simulink model "elevatorMod"  (R2020a)
settings: Solver=VariableStepAuto  StartTime=0.0  StopTime=inf  RelTol=1e-3
PreLoadFcn:
  | slplc.api.loadDataTypes;
undefined symbols (not defined in the file): BOOL, DINT, INT, slplc
libraries: simulink x1
(part 19 of 39)

== system elevatorMod/PLCControllerSuite/__Logic/Task/Program/__Logic/XIC35/Instruction_Enable ==
  Rung-condition-in : Inport  OutDataTypeStr=BOOL
  Enable : EnablePort
  Logical Operator : Logic  OutDataTypeStr=BOOL
  __CoreVarRead : Subsystem  Tag=CoreVarReadBlock  DisableCoverage=on  TreatAsAtomicUnit=on  mask{PLCBlockType=CoreVarRead}
      mask init:
      | slplc.callbacks.initCoreVariable(gcb, 'read');
      mask Help: web([docroot '/plccoder/ref/__corevarread' '.html']);
      mask DialogControl PLCBlockTitle Prompt: Core Variable Read
  Rung-condition-out : Outport  VectorParamsAs1DForOutWhenUnconnected=off
  wires:
  __CoreVarRead/1(y) -> Logical Operator/2  "DataBit"
  Logical Operator/1 -> Rung-condition-out/1  "Rung-condition-out"
  Rung-condition-in/1 -> Logical Operator/1  "Rung-condition-in"

== system elevatorMod/PLCControllerSuite/__Logic/Task/Program/__Logic/XIC35/RungInOverride ==
  In1 : Inport
  AND : Logic  AllPortsSameDT=off  OutDataTypeStr=boolean
  ForceRungInFalseRead : Subsystem  DisableCoverage=on  TreatAsAtomicUnit=on  mask{PLCLabelTag=_Force_RungIn_False, PLCBlockType=ForceRungInFalseRead}
      mask prompts: PLCLabelTag "Label Tag:"
      mask init:
      | block = gcb;
      | maskObj = Simulink.Mask.get(block);
      | maskObj.Display = sprintf('disp(''%s'');', PLCLabelTag);
      mask Help: web([docroot '/plccoder/ref/forcerunginfalseread' '.html']);
      mask DialogControl PLCBlockTitle Prompt: Force Rung-In False Read
      mask Display: disp('_Force_RungIn_False');
  NOT : Logic  Operator=NOT  IconShape=distinctive  AllPortsSameDT=off  OutDataTypeStr=boolean
  Out1 : Outport  VectorParamsAs1DForOutWhenUnconnected=off
  wires:
  NOT/1 -> AND/1
  ForceRungInFalseRead/1(Out1) -> NOT/1
  In1/1 -> AND/2
  AND/1 -> Out1/1

== system elevatorMod/PLCControllerSuite/__Logic/Task/Program/__Logic/XIC35/__CoreVarRead ==
  DataRead : DataStoreRead  DataStoreName=xxx_PLC_VAR_F2PBHold
  y : Outport  VectorParamsAs1DForOutWhenUnconnected=off
  wires:
  DataRead/1 -> y/1

== system elevatorMod/PLCControllerSuite/__Logic/Task/Program/__Logic/XIC36/BlockEnableRead ==
  __CoreLabelRead : Subsystem  Tag=CoreVarReadBlock  DisableCoverage=on  TreatAsAtomicUnit=on  mask{PLCBlockType=CoreLabelRead}
      mask init:
      | slplc.callbacks.initRoutineLabelRead(gcb);
      mask Help: web([docroot '/plccoder/ref/__corelabelread' '.html']);
      mask DialogControl PLCBlockTitle Prompt: Core Label Read
  Out1 : Outport  VectorParamsAs1DForOutWhenUnconnected=off
  wires:
  __CoreLabelRead/1(Out1) -> Out1/1

== system elevatorMod/PLCControllerSuite/__Logic/Task/Program/__Logic/XIC36/Instruction_Enable ==
  Rung-condition-in : Inport  OutDataTypeStr=BOOL
  Enable : EnablePort
  Logical Operator : Logic  OutDataTypeStr=BOOL
  __CoreVarRead : Subsystem  Tag=CoreVarReadBlock  DisableCoverage=on  TreatAsAtomicUnit=on  mask{PLCBlockType=CoreVarRead}
      mask init:
      | slplc.callbacks.initCoreVariable(gcb, 'read');
      mask Help: web([docroot '/plccoder/ref/__corevarread' '.html']);
      mask DialogControl PLCBlockTitle Prompt: Core Variable Read
  Rung-condition-out : Outport  VectorParamsAs1DForOutWhenUnconnected=off
  wires:
  Rung-condition-in/1 -> Logical Operator/1  "Rung-condition-in"
  Logical Operator/1 -> Rung-condition-out/1  "Rung-condition-out"
  __CoreVarRead/1(y) -> Logical Operator/2  "DataBit"

== system elevatorMod/PLCControllerSuite/__Logic/Task/Program/__Logic/XIC36/RungInOverride ==
  In1 : Inport
  AND : Logic  AllPortsSameDT=off  OutDataTypeStr=boolean
  ForceRungInFalseRead : Subsystem  DisableCoverage=on  TreatAsAtomicUnit=on  mask{PLCLabelTag=_Force_RungIn_False, PLCBlockType=ForceRungInFalseRead}
      mask prompts: PLCLabelTag "Label Tag:"
      mask init:
      | block = gcb;
      | maskObj = Simulink.Mask.get(block);
      | maskObj.Display = sprintf('disp(''%s'');', PLCLabelTag);
      mask Help: web([docroot '/plccoder/ref/forcerunginfalseread' '.html']);
      mask DialogControl PLCBlockTitle Prompt: Force Rung-In False Read
      mask Display: disp('_Force_RungIn_False');
  NOT : Logic  Operator=NOT  IconShape=distinctive  AllPortsSameDT=off  OutDataTypeStr=boolean
  Out1 : Outport  VectorParamsAs1DForOutWhenUnconnected=off
  wires:
  AND/1 -> Out1/1
  In1/1 -> AND/2
  ForceRungInFalseRead/1(Out1) -> NOT/1
  NOT/1 -> AND/1

== system elevatorMod/PLCControllerSuite/__Logic/Task/Program/__Logic/XIC36/__CoreVarRead ==
  DataRead : DataStoreRead  DataStoreName=xxx_PLC_VAR_F3DownBHold
  y : Outport  VectorParamsAs1DForOutWhenUnconnected=off
  wires:
  DataRead/1 -> y/1

== system elevatorMod/PLCControllerSuite/__Logic/Task/Program/__Logic/XIC37/BlockEnableRead ==
  __CoreLabelRead : Subsystem  Tag=CoreVarReadBlock  DisableCoverage=on  TreatAsAtomicUnit=on  mask{PLCBlockType=CoreLabelRead}
      mask init:
      | slplc.callbacks.initRoutineLabelRead(gcb);
      mask Help: web([docroot '/plccoder/ref/__corelabelread' '.html']);
      mask DialogControl PLCBlockTitle Prompt: Core Label Read
  Out1 : Outport  VectorParamsAs1DForOutWhenUnconnected=off
  wires:
  __CoreLabelRead/1(Out1) -> Out1/1

== system elevatorMod/PLCControllerSuite/__Logic/Task/Program/__Logic/XIC37/Instruction_Enable ==
  Rung-condition-in : Inport  OutDataTypeStr=BOOL
  Enable : EnablePort
  Logical Operator : Logic  OutDataTypeStr=BOOL
  __CoreVarRead : Subsystem  Tag=CoreVarReadBlock  DisableCoverage=on  TreatAsAtomicUnit=on  mask{PLCBlockType=CoreVarRead}
      mask init:
      | slplc.callbacks.initCoreVariable(gcb, 'read');
      mask Help: web([docroot '/plccoder/ref/__corevarread' '.html']);
      mask DialogControl PLCBlockTitle Prompt: Core Variable Read
  Rung-condition-out : Outport  VectorParamsAs1DForOutWhenUnconnected=off
  wires:
  Rung-condition-in/1 -> Logical Operator/1  "Rung-condition-in"
  Logical Operator/1 -> Rung-condition-out/1  "Rung-condition-out"
  __CoreVarRead/1(y) -> Logical Operator/2  "DataBit"

== system elevatorMod/PLCControllerSuite/__Logic/Task/Program/__Logic/XIC37/RungInOverride ==
  In1 : Inport
  AND : Logic  AllPortsSameDT=off  OutDataTypeStr=boolean
  ForceRungInFalseRead : Subsystem  DisableCoverage=on  TreatAsAtomicUnit=on  mask{PLCLabelTag=_Force_RungIn_False, PLCBlockType=ForceRungInFalseRead}
      mask prompts: PLCLabelTag "Label Tag:"
      mask init:
      | block = gcb;
      | maskObj = Simulink.Mask.get(block);
      | maskObj.Display = sprintf('disp(''%s'');', PLCLabelTag);
      mask Help: web([docroot '/plccoder/ref/forcerunginfalseread' '.html']);
      mask DialogControl PLCBlockTitle Prompt: Force Rung-In False Read
      mask Display: disp('_Force_RungIn_False');
  NOT : Logic  Operator=NOT  IconShape=distinctive  AllPortsSameDT=off  OutDataTypeStr=boolean
  Out1 : Outport  VectorParamsAs1DForOutWhenUnconnected=off
  wires:
  AND/1 -> Out1/1
  In1/1 -> AND/2
  ForceRungInFalseRead/1(Out1) -> NOT/1
  NOT/1 -> AND/1

== system elevatorMod/PLCControllerSuite/__Logic/Task/Program/__Logic/XIC37/__CoreVarRead ==
  DataRead : DataStoreRead  DataStoreName=xxx_PLC_VAR_F2PBHold
  y : Outport  VectorParamsAs1DForOutWhenUnconnected=off
  wires:
  DataRead/1 -> y/1

== system elevatorMod/PLCControllerSuite/__Logic/Task/Program/__Logic/XIC38/BlockEnableRead ==
  __CoreLabelRead : Subsystem  Tag=CoreVarReadBlock  DisableCoverage=on  TreatAsAtomicUnit=on  mask{PLCBlockType=CoreLabelRead}
      mask init:
      | slplc.callbacks.initRoutineLabelRead(gcb);
      mask Help: web([docroot '/plccoder/ref/__corelabelread' '.html']);
      mask DialogControl PLCBlockTitle Prompt: Core Label Read
  Out1 : Outport  VectorParamsAs1DForOutWhenUnconnected=off
  wires:
  __CoreLabelRead/1(Out1) -> Out1/1

== system elevatorMod/PLCControllerSuite/__Logic/Task/Program/__Logic/XIC38/Instruction_Enable ==
  Rung-condition-in : Inport  OutDataTypeStr=BOOL
  Enable : EnablePort
  Logical Operator : Logic  OutDataTypeStr=BOOL
  __CoreVarRead : Subsystem  Tag=CoreVarReadBlock  DisableCoverage=on  TreatAsAtomicUnit=on  mask{PLCBlockType=CoreVarRead}
      mask init:
      | slplc.callbacks.initCoreVariable(gcb, 'read');
      mask Help: web([docroot '/plccoder/ref/__corevarread' '.html']);
      mask DialogControl PLCBlockTitle Prompt: Core Variable Read
  Rung-condition-out : Outport  VectorParamsAs1DForOutWhenUnconnected=off
  wires:
  __CoreVarRead/1(y) -> Logical Operator/2  "DataBit"
  Logical Operator/1 -> Rung-condition-out/1  "Rung-condition-out"
  Rung-condition-in/1 -> Logical Operator/1  "Rung-condition-in"

== system elevatorMod/PLCControllerSuite/__Logic/Task/Program/__Logic/XIC38/RungInOverride ==
  In1 : Inport
  AND : Logic  AllPortsSameDT=off  OutDataTypeStr=boolean
  ForceRungInFalseRead : Subsystem  DisableCoverage=on  TreatAsAtomicUnit=on  mask{PLCLabelTag=_Force_RungIn_False, PLCBlockType=ForceRungInFalseRead}
      mask prompts: PLCLabelTag "Label Tag:"
      mask init:
      | block = gcb;
      | maskObj = Simulink.Mask.get(block);
      | maskObj.Display = sprintf('disp(''%s'');', PLCLabelTag);
      mask Help: web([docroot '/plccoder/ref/forcerunginfalseread' '.html']);
      mask DialogControl PLCBlockTitle Prompt: Force Rung-In False Read
      mask Display: disp('_Force_RungIn_False');
  NOT : Logic  Operator=NOT  IconShape=distinctive  AllPortsSameDT=off  OutDataTypeStr=boolean
  Out1 : Outport  VectorParamsAs1DForOutWhenUnconnected=off
  wires:
  NOT/1 -> AND/1
  ForceRungInFalseRead/1(Out1) -> NOT/1
  In1/1 -> AND/2
  AND/1 -> Out1/1

== system elevatorMod/PLCControllerSuite/__Logic/Task/Program/__Logic/XIC38/__CoreVarRead ==
  DataRead : DataStoreRead  DataStoreName=xxx_PLC_VAR_MTRON
  y : Outport  VectorParamsAs1DForOutWhenUnconnected=off
  wires:
  DataRead/1 -> y/1

== system elevatorMod/PLCControllerSuite/__Logic/Task/Program/__Logic/XIC39/BlockEnableRead ==
  __CoreLabelRead : Subsystem  Tag=CoreVarReadBlock  DisableCoverage=on  TreatAsAtomicUnit=on  mask{PLCBlockType=CoreLabelRead}
      mask init:
      | slplc.callbacks.initRoutineLabelRead(gcb);
      mask Help: web([docroot '/plccoder/ref/__corelabelread' '.html']);
      mask DialogControl PLCBlockTitle Prompt: Core Label Read
  Out1 : Outport  VectorParamsAs1DForOutWhenUnconnected=off
  wires:
  __CoreLabelRead/1(Out1) -> Out1/1

== system elevatorMod/PLCControllerSuite/__Logic/Task/Program/__Logic/XIC39/Instruction_Enable ==
  Rung-condition-in : Inport  OutDataTypeStr=BOOL
  Enable : EnablePort
  Logical Operator : Logic  OutDataTypeStr=BOOL
  __CoreVarRead : Subsystem  Tag=CoreVarReadBlock  DisableCoverage=on  TreatAsAtomicUnit=on  mask{PLCBlockType=CoreVarRead}
      mask init:
      | slplc.callbacks.initCoreVariable(gcb, 'read');
      mask Help: web([docroot '/plccoder/ref/__corevarread' '.html']);
      mask DialogControl PLCBlockTitle Prompt: Core Variable Read
  Rung-condition-out : Outport  VectorParamsAs1DForOutWhenUnconnected=off
  wires:
  Rung-condition-in/1 -> Logical Operator/1  "Rung-condition-in"
  Logical Operator/1 -> Rung-condition-out/1  "Rung-condition-out"
  __CoreVarRead/1(y) -> Logical Operator/2  "DataBit"

== system elevatorMod/PLCControllerSuite/__Logic/Task/Program/__Logic/XIC39/RungInOverride ==
  In1 : Inport
  AND : Logic  AllPortsSameDT=off  OutDataTypeStr=boolean
  ForceRungInFalseRead : Subsystem  DisableCoverage=on  TreatAsAtomicUnit=on  mask{PLCLabelTag=_Force_RungIn_False, PLCBlockType=ForceRungInFalseRead}
      mask prompts: PLCLabelTag "Label Tag:"
      mask init:
      | block = gcb;
      | maskObj = Simulink.Mask.get(block);
      | maskObj.Display = sprintf('disp(''%s'');', PLCLabelTag);
      mask Help: web([docroot '/plccoder/ref/forcerunginfalseread' '.html']);
      mask DialogControl PLCBlockTitle Prompt: Force Rung-In False Read
      mask Display: disp('_Force_RungIn_False');
  NOT : Logic  Operator=NOT  IconShape=distinctive  AllPortsSameDT=off  OutDataTypeStr=boolean
  Out1 : Outport  VectorParamsAs1DForOutWhenUnconnected=off
  wires:
  AND/1 -> Out1/1
  In1/1 -> AND/2
  ForceRungInFalseRead/1(Out1) -> NOT/1
  NOT/1 -> AND/1

== system elevatorMod/PLCControllerSuite/__Logic/Task/Program/__Logic/XIC39/__CoreVarRead ==
  DataRead : DataStoreRead  DataStoreName=xxx_PLC_VAR_RMPUPTRG
  y : Outport  VectorParamsAs1DForOutWhenUnconnected=off
  wires:
  DataRead/1 -> y/1

== system elevatorMod/PLCControllerSuite/__Logic/Task/Program/__Logic/XIC4/BlockEnableRead ==
  __CoreLabelRead : Subsystem  Tag=CoreVarReadBlock  DisableCoverage=on  TreatAsAtomicUnit=on  mask{PLCBlockType=CoreLabelRead}
      mask init:
      | slplc.callbacks.initRoutineLabelRead(gcb);
      mask Help: web([docroot '/plccoder/ref/__corelabelread' '.html']);
      mask DialogControl PLCBlockTitle Prompt: Core Label Read
  Out1 : Outport  VectorParamsAs1DForOutWhenUnconnected=off
  wires:
  __CoreLabelRead/1(Out1) -> Out1/1

== system elevatorMod/PLCControllerSuite/__Logic/Task/Program/__Logic/XIC4/Instruction_Enable ==
  Rung-condition-in : Inport  OutDataTypeStr=BOOL
  Enable : EnablePort
  Logical Operator : Logic  OutDataTypeStr=BOOL
  __CoreVarRead : Subsystem  Tag=CoreVarReadBlock  DisableCoverage=on  TreatAsAtomicUnit=on  mask{PLCBlockType=CoreVarRead}
      mask init:
      | slplc.callbacks.initCoreVariable(gcb, 'read');
      mask Help: web([docroot '/plccoder/ref/__corevarread' '.html']);
      mask DialogControl PLCBlockTitle Prompt: Core Variable Read
  Rung-condition-out : Outport  VectorParamsAs1DForOutWhenUnconnected=off
  wires:
  Rung-condition-in/1 -> Logical Operator/1  "Rung-condition-in"
  Logical Operator/1 -> Rung-condition-out/1  "Rung-condition-out"
  __CoreVarRead/1(y) -> Logical Operator/2  "DataBit"

== system elevatorMod/PLCControllerSuite/__Logic/Task/Program/__Logic/XIC4/RungInOverride ==
  In1 : Inport
  AND : Logic  AllPortsSameDT=off  OutDataTypeStr=boolean
  ForceRungInFalseRead : Subsystem  DisableCoverage=on  TreatAsAtomicUnit=on  mask{PLCLabelTag=_Force_RungIn_False, PLCBlockType=ForceRungInFalseRead}
      mask prompts: PLCLabelTag "Label Tag:"
      mask init:
      | block = gcb;
      | maskObj = Simulink.Mask.get(block);
      | maskObj.Display = sprintf('disp(''%s'');', PLCLabelTag);
      mask Help: web([docroot '/plccoder/ref/forcerunginfalseread' '.html']);
      mask DialogControl PLCBlockTitle Prompt: Force Rung-In False Read
      mask Display: disp('_Force_RungIn_False');
  NOT : Logic  Operator=NOT  IconShape=distinctive  AllPortsSameDT=off  OutDataTypeStr=boolean
  Out1 : Outport  VectorParamsAs1DForOutWhenUnconnected=off
  wires:
  AND/1 -> Out1/1
  In1/1 -> AND/2
  ForceRungInFalseRead/1(Out1) -> NOT/1
  NOT/1 -> AND/1

== system elevatorMod/PLCControllerSuite/__Logic/Task/Program/__Logic/XIC4/__CoreVarRead ==
  DataRead : DataStoreRead  DataStoreName=xxx_PLC_VAR_F1PBHold
  y : Outport  VectorParamsAs1DForOutWhenUnconnected=off
  wires:
  DataRead/1 -> y/1

== system elevatorMod/PLCControllerSuite/__Logic/Task/Program/__Logic/XIC40/BlockEnableRead ==
  __CoreLabelRead : Subsystem  Tag=CoreVarReadBlock  DisableCoverage=on  TreatAsAtomicUnit=on  mask{PLCBlockType=CoreLabelRead}
      mask init:
      | slplc.callbacks.initRoutineLabelRead(gcb);
      mask Help: web([docroot '/plccoder/ref/__corelabelread' '.html']);
      mask DialogControl PLCBlockTitle Prompt: Core Label Read
  Out1 : Outport  VectorParamsAs1DForOutWhenUnconnected=off
  wires:
  __CoreLabelRead/1(Out1) -> Out1/1

== system elevatorMod/PLCControllerSuite/__Logic/Task/Program/__Logic/XIC40/Instruction_Enable ==
  Rung-condition-in : Inport  OutDataTypeStr=BOOL
  Enable : EnablePort
  Logical Operator : Logic  OutDataTypeStr=BOOL
  __CoreVarRead : Subsystem  Tag=CoreVarReadBlock  DisableCoverage=on  TreatAsAtomicUnit=on  mask{PLCBlockType=CoreVarRead}
      mask init:
      | slplc.callbacks.initCoreVariable(gcb, 'read');
      mask Help: web([docroot '/plccoder/ref/__corevarread' '.html']);
      mask DialogControl PLCBlockTitle Prompt: Core Variable Read
  Rung-condition-out : Outport  VectorParamsAs1DForOutWhenUnconnected=off
  wires:
  __CoreVarRead/1(y) -> Logical Operator/2  "DataBit"
  Logical Operator/1 -> Rung-condition-out/1  "Rung-condition-out"
  Rung-condition-in/1 -> Logical Operator/1  "Rung-condition-in"

== system elevatorMod/PLCControllerSuite/__Logic/Task/Program/__Logic/XIC40/RungInOverride ==
  In1 : Inport
  AND : Logic  AllPortsSameDT=off  OutDataTypeStr=boolean
  ForceRungInFalseRead : Subsystem  DisableCoverage=on  TreatAsAtomicUnit=on  mask{PLCLabelTag=_Force_RungIn_False, PLCBlockType=ForceRungInFalseRead}
      mask prompts: PLCLabelTag "Label Tag:"
      mask init:
      | block = gcb;
      | maskObj = Simulink.Mask.get(block);
      | maskObj.Display = sprintf('disp(''%s'');', PLCLabelTag);
      mask Help: web([docroot '/plccoder/ref/forcerunginfalseread' '.html']);
      mask DialogControl PLCBlockTitle Prompt: Force Rung-In False Read
      mask Display: disp('_Force_RungIn_False');
  NOT : Logic  Operator=NOT  IconShape=distinctive  AllPortsSameDT=off  OutDataTypeStr=boolean
  Out1 : Outport  VectorParamsAs1DForOutWhenUnconnected=off
  wires:
  NOT/1 -> AND/1
  ForceRungInFalseRead/1(Out1) -> NOT/1
  In1/1 -> AND/2
  AND/1 -> Out1/1

== system elevatorMod/PLCControllerSuite/__Logic/Task/Program/__Logic/XIC40/__CoreVarRead ==
  DataRead : DataStoreRead  DataStoreName=xxx_PLC_VAR_RMPUP
  y : Outport  VectorParamsAs1DForOutWhenUnconnected=off
  wires:
  DataRead/1 -> y/1

== system elevatorMod/PLCControllerSuite/__Logic/Task/Program/__Logic/XIC41/BlockEnableRead ==
  __CoreLabelRead : Subsystem  Tag=CoreVarReadBlock  DisableCoverage=on  TreatAsAtomicUnit=on  mask{PLCBlockType=CoreLabelRead}
      mask init:
      | slplc.callbacks.initRoutineLabelRead(gcb);
      mask Help: web([docroot '/plccoder/ref/__corelabelread' '.html']);
      mask DialogControl PLCBlockTitle Prompt: Core Label Read
  Out1 : Outport  VectorParamsAs1DForOutWhenUnconnected=off
  wires:
  __CoreLabelRead/1(Out1) -> Out1/1

== system elevatorMod/PLCControllerSuite/__Logic/Task/Program/__Logic/XIC41/Instruction_Enable ==
  Rung-condition-in : Inport  OutDataTypeStr=BOOL
  Enable : EnablePort
  Logical Operator : Logic  OutDataTypeStr=BOOL
  __CoreVarRead : Subsystem  Tag=CoreVarReadBlock  DisableCoverage=on  TreatAsAtomicUnit=on  mask{PLCBlockType=CoreVarRead}
      mask init:
      | slplc.callbacks.initCoreVariable(gcb, 'read');
      mask Help: web([docroot '/plccoder/ref/__corevarread' '.html']);
      mask DialogControl PLCBlockTitle Prompt: Core Variable Read
  Rung-condition-out : Outport  VectorParamsAs1DForOutWhenUnconnected=off
  wires:
  __CoreVarRead/1(y) -> Logical Operator/2  "DataBit"
  Logical Operator/1 -> Rung-condition-out/1  "Rung-condition-out"
  Rung-condition-in/1 -> Logical Operator/1  "Rung-condition-in"

== system elevatorMod/PLCControllerSuite/__Logic/Task/Program/__Logic/XIC41/RungInOverride ==
  In1 : Inport
  AND : Logic  AllPortsSameDT=off  OutDataTypeStr=boolean
  ForceRungInFalseRead : Subsystem  DisableCoverage=on  TreatAsAtomicUnit=on  mask{PLCLabelTag=_Force_RungIn_False, PLCBlockType=ForceRungInFalseRead}
      mask prompts: PLCLabelTag "Label Tag:"
      mask init:
      | block = gcb;
      | maskObj = Simulink.Mask.get(block);
      | maskObj.Display = sprintf('disp(''%s'');', PLCLabelTag);
      mask Help: web([docroot '/plccoder/ref/forcerunginfalseread' '.html']);
      mask DialogControl PLCBlockTitle Prompt: Force Rung-In False Read
      mask Display: disp('_Force_RungIn_False');
  NOT : Logic  Operator=NOT  IconShape=distinctive  AllPortsSameDT=off  OutDataTypeStr=boolean
  Out1 : Outport  VectorParamsAs1DForOutWhenUnconnected=off
  wires:
  NOT/1 -> AND/1
  ForceRungInFalseRead/1(Out1) -> NOT/1
  In1/1 -> AND/2
  AND/1 -> Out1/1

== system elevatorMod/PLCControllerSuite/__Logic/Task/Program/__Logic/XIC41/__CoreVarRead ==
  DataRead : DataStoreRead  DataStoreName=xxx_PLC_VAR_SENCHK
  y : Outport  VectorParamsAs1DForOutWhenUnconnected=off
  wires:
  DataRead/1 -> y/1

== system elevatorMod/PLCControllerSuite/__Logic/Task/Program/__Logic/XIC42/BlockEnableRead ==
  __CoreLabelRead : Subsystem  Tag=CoreVarReadBlock  DisableCoverage=on  TreatAsAtomicUnit=on  mask{PLCBlockType=CoreLabelRead}
      mask init:
      | slplc.callbacks.initRoutineLabelRead(gcb);
      mask Help: web([docroot '/plccoder/ref/__corelabelread' '.html']);
      mask DialogControl PLCBlockTitle Prompt: Core Label Read
  Out1 : Outport  VectorParamsAs1DForOutWhenUnconnected=off
  wires:
  __CoreLabelRead/1(Out1) -> Out1/1

== system elevatorMod/PLCControllerSuite/__Logic/Task/Program/__Logic/XIC42/Instruction_Enable ==
  Rung-condition-in : Inport  OutDataTypeStr=BOOL
  Enable : EnablePort
  Logical Operator : Logic  OutDataTypeStr=BOOL
  __CoreVarRead : Subsystem  Tag=CoreVarReadBlock  DisableCoverage=on  TreatAsAtomicUnit=on  mask{PLCBlockType=CoreVarRead}
      mask init:
      | slplc.callbacks.initCoreVariable(gcb, 'read');
      mask Help: web([docroot '/plccoder/ref/__corevarread' '.html']);
      mask DialogControl PLCBlockTitle Prompt: Core Variable Read
  Rung-condition-out : Outport  VectorParamsAs1DForOutWhenUnconnected=off
  wires:
  Rung-condition-in/1 -> Logical Operator/1  "Rung-condition-in"
  Logical Operator/1 -> Rung-condition-out/1  "Rung-condition-out"
  __CoreVarRead/1(y) -> Logical Operator/2  "DataBit"

== system elevatorMod/PLCControllerSuite/__Logic/Task/Program/__Logic/XIC42/RungInOverride ==
  In1 : Inport
  AND : Logic  AllPortsSameDT=off  OutDataTypeStr=boolean
  ForceRungInFalseRead : Subsystem  DisableCoverage=on  TreatAsAtomicUnit=on  mask{PLCLabelTag=_Force_RungIn_False, PLCBlockType=ForceRungInFalseRead}
      mask prompts: PLCLabelTag "Label Tag:"
      mask init:
      | block = gcb;
      | maskObj = Simulink.Mask.get(block);
      | maskObj.Display = sprintf('disp(''%s'');', PLCLabelTag);
      mask Help: web([docroot '/plccoder/ref/forcerunginfalseread' '.html']);
      mask DialogControl PLCBlockTitle Prompt: Force Rung-In False Read
      mask Display: disp('_Force_RungIn_False');
  NOT : Logic  Operator=NOT  IconShape=distinctive  AllPortsSameDT=off  OutDataTypeStr=boolean
  Out1 : Outport  VectorParamsAs1DForOutWhenUnconnected=off
  wires:
  AND/1 -> Out1/1
  In1/1 -> AND/2
  ForceRungInFalseRead/1(Out1) -> NOT/1
  NOT/1 -> AND/1

== system elevatorMod/PLCControllerSuite/__Logic/Task/Program/__Logic/XIC42/__CoreVarRead ==
  DataRead : DataStoreRead  DataStoreName=xxx_PLC_VAR_StartHold
  y : Outport  VectorParamsAs1DForOutWhenUnconnected=off
  wires:
  DataRead/1 -> y/1

== system elevatorMod/PLCControllerSuite/__Logic/Task/Program/__Logic/XIC43/BlockEnableRead ==
  __CoreLabelRead : Subsystem  Tag=CoreVarReadBlock  DisableCoverage=on  TreatAsAtomicUnit=on  mask{PLCBlockType=CoreLabelRead}
      mask init:
      | slplc.callbacks.initRoutineLabelRead(gcb);
      mask Help: web([docroot '/plccoder/ref/__corelabelread' '.html']);
      mask DialogControl PLCBlockTitle Prompt: Core Label Read
  Out1 : Outport  VectorParamsAs1DForOutWhenUnconnected=off
  wires:
  __CoreLabelRead/1(Out1) -> Out1/1

== system elevatorMod/PLCControllerSuite/__Logic/Task/Program/__Logic/XIC43/Instruction_Enable ==
  Rung-condition-in : Inport  OutDataTypeStr=BOOL
  Enable : EnablePort
  Logical Operator : Logic  OutDataTypeStr=BOOL
  __CoreVarRead : Subsystem  Tag=CoreVarReadBlock  DisableCoverage=on  TreatAsAtomicUnit=on  mask{PLCBlockType=CoreVarRead}
      mask init:
      | slplc.callbacks.initCoreVariable(gcb, 'read');
      mask Help: web([docroot '/plccoder/ref/__corevarread' '.html']);
      mask DialogControl PLCBlockTitle Prompt: Core Variable Read
  Rung-condition-out : Outport  VectorParamsAs1DForOutWhenUnconnected=off
  wires:
  Rung-condition-in/1 -> Logical Operator/1  "Rung-condition-in"
  Logical Operator/1 -> Rung-condition-out/1  "Rung-condition-out"
  __CoreVarRead/1(y) -> Logical Operator/2  "DataBit"

== system elevatorMod/PLCControllerSuite/__Logic/Task/Program/__Logic/XIC43/RungInOverride ==
  In1 : Inport
  AND : Logic  AllPortsSameDT=off  OutDataTypeStr=boolean
  ForceRungInFalseRead : Subsystem  DisableCoverage=on  TreatAsAtomicUnit=on  mask{PLCLabelTag=_Force_RungIn_False, PLCBlockType=ForceRungInFalseRead}
      mask prompts: PLCLabelTag "Label Tag:"
      mask init:
      | block = gcb;
      | maskObj = Simulink.Mask.get(block);
      | maskObj.Display = sprintf('disp(''%s'');', PLCLabelTag);
      mask Help: web([docroot '/plccoder/ref/forcerunginfalseread' '.html']);
      mask DialogControl PLCBlockTitle Prompt: Force Rung-In False Read
      mask Display: disp('_Force_RungIn_False');
  NOT : Logic  Operator=NOT  IconShape=distinctive  AllPortsSameDT=off  OutDataTypeStr=boolean
  Out1 : Outport  VectorParamsAs1DForOutWhenUnconnected=off
  wires:
  AND/1 -> Out1/1
  In1/1 -> AND/2
  ForceRungInFalseRead/1(Out1) -> NOT/1
  NOT/1 -> AND/1

== system elevatorMod/PLCControllerSuite/__Logic/Task/Program/__Logic/XIC43/__CoreVarRead ==
  DataRead : DataStoreRead  DataStoreName=xxx_PLC_VAR_TempS3LUp
  y : Outport  VectorParamsAs1DForOutWhenUnconnected=off
  wires:
  DataRead/1 -> y/1

== system elevatorMod/PLCControllerSuite/__Logic/Task/Program/__Logic/XIC44/BlockEnableRead ==
  __CoreLabelRead : Subsystem  Tag=CoreVarReadBlock  DisableCoverage=on  TreatAsAtomicUnit=on  mask{PLCBlockType=CoreLabelRead}
      mask init:
      | slplc.callbacks.initRoutineLabelRead(gcb);
      mask Help: web([docroot '/plccoder/ref/__corelabelread' '.html']);
      mask DialogControl PLCBlockTitle Prompt: Core Label Read
  Out1 : Outport  VectorParamsAs1DForOutWhenUnconnected=off
  wires:
  __CoreLabelRead/1(Out1) -> Out1/1

== system elevatorMod/PLCControllerSuite/__Logic/Task/Program/__Logic/XIC44/Instruction_Enable ==
  Rung-condition-in : Inport  OutDataTypeStr=BOOL
  Enable : EnablePort
  Logical Operator : Logic  OutDataTypeStr=BOOL
  __CoreVarRead : Subsystem  Tag=CoreVarReadBlock  DisableCoverage=on  TreatAsAtomicUnit=on  mask{PLCBlockType=CoreVarRead}
      mask init:
      | slplc.callbacks.initCoreVariable(gcb, 'read');
      mask Help: web([docroot '/plccoder/ref/__corevarread' '.html']);
      mask DialogControl PLCBlockTitle Prompt: Core Variable Read
  Rung-condition-out : Outport  VectorParamsAs1DForOutWhenUnconnected=off
  wires:
  __CoreVarRead/1(y) -> Logical Operator/2  "DataBit"
  Logical Operator/1 -> Rung-condition-out/1  "Rung-condition-out"
  Rung-condition-in/1 -> Logical Operator/1  "Rung-condition-in"

== system elevatorMod/PLCControllerSuite/__Logic/Task/Program/__Logic/XIC44/RungInOverride ==
  In1 : Inport
  AND : Logic  AllPortsSameDT=off  OutDataTypeStr=boolean
  ForceRungInFalseRead : Subsystem  DisableCoverage=on  TreatAsAtomicUnit=on  mask{PLCLabelTag=_Force_RungIn_False, PLCBlockType=ForceRungInFalseRead}
      mask prompts: PLCLabelTag "Label Tag:"
      mask init:
      | block = gcb;
      | maskObj = Simulink.Mask.get(block);
      | maskObj.Display = sprintf('disp(''%s'');', PLCLabelTag);
      mask Help: web([docroot '/plccoder/ref/forcerunginfalseread' '.html']);
      mask DialogControl PLCBlockTitle Prompt: Force Rung-In False Read
      mask Display: disp('_Force_RungIn_False');
  NOT : Logic  Operator=NOT  IconShape=distinctive  AllPortsSameDT=off  OutDataTypeStr=boolean
  Out1 : Outport  VectorParamsAs1DForOutWhenUnconnected=off
  wires:
  NOT/1 -> AND/1
  ForceRungInFalseRead/1(Out1) -> NOT/1
  In1/1 -> AND/2
  AND/1 -> Out1/1

== system elevatorMod/PLCControllerSuite/__Logic/Task/Program/__Logic/XIC44/__CoreVarRead ==
  DataRead : DataStoreRead  DataStoreName=xxx_PLC_VAR_MemoryGoUp
  y : Outport  VectorParamsAs1DForOutWhenUnconnected=off
  wires:
  DataRead/1 -> y/1

== system elevatorMod/PLCControllerSuite/__Logic/Task/Program/__Logic/XIC45/BlockEnableRead ==
  __CoreLabelRead : Subsystem  Tag=CoreVarReadBlock  DisableCoverage=on  TreatAsAtomicUnit=on  mask{PLCBlockType=CoreLabelRead}
      mask init:
      | slplc.callbacks.initRoutineLabelRead(gcb);
      mask Help: web([docroot '/plccoder/ref/__corelabelread' '.html']);
      mask DialogControl PLCBlockTitle Prompt: Core Label Read
  Out1 : Outport  VectorParamsAs1DForOutWhenUnconnected=off
  wires:
  __CoreLabelRead/1(Out1) -> Out1/1

== system elevatorMod/PLCControllerSuite/__Logic/Task/Program/__Logic/XIC45/Instruction_Enable ==
  Rung-condition-in : Inport  OutDataTypeStr=BOOL
  Enable : EnablePort
  Logical Operator : Logic  OutDataTypeStr=BOOL
  __CoreVarRead : Subsystem  Tag=CoreVarReadBlock  DisableCoverage=on  TreatAsAtomicUnit=on  mask{PLCBlockType=CoreVarRead}
      mask init:
      | slplc.callbacks.initCoreVariable(gcb, 'read');
      mask Help: web([docroot '/plccoder/ref/__corevarread' '.html']);
      mask DialogControl PLCBlockTitle Prompt: Core Variable Read
  Rung-condition-out : Outport  VectorParamsAs1DForOutWhenUnconnected=off
  wires:
  Rung-condition-in/1 -> Logical Operator/1  "Rung-condition-in"
  Logical Operator/1 -> Rung-condition-out/1  "Rung-condition-out"
  __CoreVarRead/1(y) -> Logical Operator/2  "DataBit"

== system elevatorMod/PLCControllerSuite/__Logic/Task/Program/__Logic/XIC45/RungInOverride ==
  In1 : Inport
  AND : Logic  AllPortsSameDT=off  OutDataTypeStr=boolean
  ForceRungInFalseRead : Subsystem  DisableCoverage=on  TreatAsAtomicUnit=on  mask{PLCLabelTag=_Force_RungIn_False, PLCBlockType=ForceRungInFalseRead}
      mask prompts: PLCLabelTag "Label Tag:"
      mask init:
      | block = gcb;
      | maskObj = Simulink.Mask.get(block);
      | maskObj.Display = sprintf('disp(''%s'');', PLCLabelTag);
      mask Help: web([docroot '/plccoder/ref/forcerunginfalseread' '.html']);
      mask DialogControl PLCBlockTitle Prompt: Force Rung-In False Read
      mask Display: disp('_Force_RungIn_False');
  NOT : Logic  Operator=NOT  IconShape=distinctive  AllPortsSameDT=off  OutDataTypeStr=boolean
  Out1 : Outport  VectorParamsAs1DForOutWhenUnconnected=off
  wires:
  AND/1 -> Out1/1
  In1/1 -> AND/2
  ForceRungInFalseRead/1(Out1) -> NOT/1
  NOT/1 -> AND/1

== system elevatorMod/PLCControllerSuite/__Logic/Task/Program/__Logic/XIC45/__CoreVarRead ==
  DataRead : DataStoreRead  DataStoreName=xxx_PLC_VAR_StartHold
  y : Outport  VectorParamsAs1DForOutWhenUnconnected=off
  wires:
  DataRead/1 -> y/1

== system elevatorMod/PLCControllerSuite/__Logic/Task/Program/__Logic/XIC46/BlockEnableRead ==
  __CoreLabelRead : Subsystem  Tag=CoreVarReadBlock  DisableCoverage=on  TreatAsAtomicUnit=on  mask{PLCBlockType=CoreLabelRead}
      mask init:
      | slplc.callbacks.initRoutineLabelRead(gcb);
      mask Help: web([docroot '/plccoder/ref/__corelabelread' '.html']);
      mask DialogControl PLCBlockTitle Prompt: Core Label Read
  Out1 : Outport  VectorParamsAs1DForOutWhenUnconnected=off
  wires:
  __CoreLabelRead/1(Out1) -> Out1/1

== system elevatorMod/PLCControllerSuite/__Logic/Task/Program/__Logic/XIC46/Instruction_Enable ==
  Rung-condition-in : Inport  OutDataTypeStr=BOOL
  Enable : EnablePort
  Logical Operator : Logic  OutDataTypeStr=BOOL
  __CoreVarRead : Subsystem  Tag=CoreVarReadBlock  DisableCoverage=on  TreatAsAtomicUnit=on  mask{PLCBlockType=CoreVarRead}
      mask init:
      | slplc.callbacks.initCoreVariable(gcb, 'read');
      mask Help: web([docroot '/plccoder/ref/__corevarread' '.html']);
      mask DialogControl PLCBlockTitle Prompt: Core Variable Read
  Rung-condition-out : Outport  VectorParamsAs1DForOutWhenUnconnected=off
  wires:
  __CoreVarRead/1(y) -> Logical Operator/2  "DataBit"
  Logical Operator/1 -> Rung-condition-out/1  "Rung-condition-out"
  Rung-condition-in/1 -> Logical Operator/1  "Rung-condition-in"

== system elevatorMod/PLCControllerSuite/__Logic/Task/Program/__Logic/XIC46/RungInOverride ==
  In1 : Inport
  AND : Logic  AllPortsSameDT=off  OutDataTypeStr=boolean
  ForceRungInFalseRead : Subsystem  DisableCoverage=on  TreatAsAtomicUnit=on  mask{PLCLabelTag=_Force_RungIn_False, PLCBlockType=ForceRungInFalseRead}
      mask prompts: PLCLabelTag "Label Tag:"
      mask init:
      | block = gcb;
      | maskObj = Simulink.Mask.get(block);
      | maskObj.Display = sprintf('disp(''%s'');', PLCLabelTag);
      mask Help: web([docroot '/plccoder/ref/forcerunginfalseread' '.html']);
      mask DialogControl PLCBlockTitle Prompt: Force Rung-In False Read
      mask Display: disp('_Force_RungIn_False');
  NOT : Logic  Operator=NOT  IconShape=distinctive  AllPortsSameDT=off  OutDataTypeStr=boolean
  Out1 : Outport  VectorParamsAs1DForOutWhenUnconnected=off
  wires:
  NOT/1 -> AND/1
  ForceRungInFalseRead/1(Out1) -> NOT/1
  In1/1 -> AND/2
  AND/1 -> Out1/1

== system elevatorMod/PLCControllerSuite/__Logic/Task/Program/__Logic/XIC46/__CoreVarRead ==
  DataRead : DataStoreRead  DataStoreName=xxx_PLC_VAR_S1H
  y : Outport  VectorParamsAs1DForOutWhenUnconnected=off
  wires:
  DataRead/1 -> y/1

== system elevatorMod/PLCControllerSuite/__Logic/Task/Program/__Logic/XIC47/BlockEnableRead ==
  __CoreLabelRead : Subsystem  Tag=CoreVarReadBlock  DisableCoverage=on  TreatAsAtomicUnit=on  mask{PLCBlockType=CoreLabelRead}
      mask init:
      | slplc.callbacks.initRoutineLabelRead(gcb);
      mask Help: web([docroot '/plccoder/ref/__corelabelread' '.html']);
      mask DialogControl PLCBlockTitle Prompt: Core Label Read
  Out1 : Outport  VectorParamsAs1DForOutWhenUnconnected=off
  wires:
  __CoreLabelRead/1(Out1) -> Out1/1

== system elevatorMod/PLCControllerSuite/__Logic/Task/Program/__Logic/XIC47/Instruction_Enable ==
  Rung-condition-in : Inport  OutDataTypeStr=BOOL
  Enable : EnablePort
  Logical Operator : Logic  OutDataTypeStr=BOOL
  __CoreVarRead : Subsystem  Tag=CoreVarReadBlock  DisableCoverage=on  TreatAsAtomicUnit=on  mask{PLCBlockType=CoreVarRead}
      mask init:
      | slplc.callbacks.initCoreVariable(gcb, 'read');
      mask Help: web([docroot '/plccoder/ref/__corevarread' '.html']);
      mask DialogControl PLCBlockTitle Prompt: Core Variable Read
  Rung-condition-out : Outport  VectorParamsAs1DForOutWhenUnconnected=off
  wires:
  Rung-condition-in/1 -> Logical Operator/1  "Rung-condition-in"
  Logical Operator/1 -> Rung-condition-out/1  "Rung-condition-out"
  __CoreVarRead/1(y) -> Logical Operator/2  "DataBit"

== system elevatorMod/PLCControllerSuite/__Logic/Task/Program/__Logic/XIC47/RungInOverride ==
  In1 : Inport
  AND : Logic  AllPortsSameDT=off  OutDataTypeStr=boolean
  ForceRungInFalseRead : Subsystem  DisableCoverage=on  TreatAsAtomicUnit=on  mask{PLCLabelTag=_Force_RungIn_False, PLCBlockType=ForceRungInFalseRead}
      mask prompts: PLCLabelTag "Label Tag:"
      mask init:
      | block = gcb;
      | maskObj = Simulink.Mask.get(block);
      | maskObj.Display = sprintf('disp(''%s'');', PLCLabelTag);
      mask Help: web([docroot '/plccoder/ref/forcerunginfalseread' '.html']);
      mask DialogControl PLCBlockTitle Prompt: Force Rung-In False Read
      mask Display: disp('_Force_RungIn_False');
  NOT : Logic  Operator=NOT  IconShape=distinctive  AllPortsSameDT=off  OutDataTypeStr=boolean
  Out1 : Outport  VectorParamsAs1DForOutWhenUnconnected=off
  wires:
  AND/1 -> Out1/1
  In1/1 -> AND/2
  ForceRungInFalseRead/1(Out1) -> NOT/1
  NOT/1 -> AND/1

== system elevatorMod/PLCControllerSuite/__Logic/Task/Program/__Logic/XIC47/__CoreVarRead ==
  DataRead : DataStoreRead  DataStoreName=xxx_PLC_VAR_S2L
  y : Outport  VectorParamsAs1DForOutWhenUnconnected=off
  wires:
  DataRead/1 -> y/1

== system elevatorMod/PLCControllerSuite/__Logic/Task/Program/__Logic/XIC48/BlockEnableRead ==
  __CoreLabelRead : Subsystem  Tag=CoreVarReadBlock  DisableCoverage=on  TreatAsAtomicUnit=on  mask{PLCBlockType=CoreLabelRead}
      mask init:
      | slplc.callbacks.initRoutineLabelRead(gcb);
      mask Help: web([docroot '/plccoder/ref/__corelabelread' '.html']);
      mask DialogControl PLCBlockTitle Prompt: Core Label Read
  Out1 : Outport  VectorParamsAs1DForOutWhenUnconnected=off
  wires:
  __CoreLabelRead/1(Out1) -> Out1/1

== system elevatorMod/PLCControllerSuite/__Logic/Task/Program/__Logic/XIC48/Instruction_Enable ==
  Rung-condition-in : Inport  OutDataTypeStr=BOOL
  Enable : EnablePort
  Logical Operator : Logic  OutDataTypeStr=BOOL
  __CoreVarRead : Subsystem  Tag=CoreVarReadBlock  DisableCoverage=on  TreatAsAtomicUnit=on  mask{PLCBlockType=CoreVarRead}
      mask init:
      | slplc.callbacks.initCoreVariable(gcb, 'read');
      mask Help: web([docroot '/plccoder/ref/__corevarread' '.html']);
      mask DialogControl PLCBlockTitle Prompt: Core Variable Read
  Rung-condition-out : Outport  VectorParamsAs1DForOutWhenUnconnected=off
  wires:
  Rung-condition-in/1 -> Logical Operator/1  "Rung-condition-in"
  Logical Operator/1 -> Rung-condition-out/1  "Rung-condition-out"
  __CoreVarRead/1(y) -> Logical Operator/2  "DataBit"

== system elevatorMod/PLCControllerSuite/__Logic/Task/Program/__Logic/XIC48/RungInOverride ==
  In1 : Inport
  AND : Logic  AllPortsSameDT=off  OutDataTypeStr=boolean
  ForceRungInFalseRead : Subsystem  DisableCoverage=on  TreatAsAtomicUnit=on  mask{PLCLabelTag=_Force_RungIn_False, PLCBlockType=ForceRungInFalseRead}
      mask prompts: PLCLabelTag "Label Tag:"
      mask init:
      | block = gcb;
      | maskObj = Simulink.Mask.get(block);
      | maskObj.Display = sprintf('disp(''%s'');', PLCLabelTag);
      mask Help: web([docroot '/plccoder/ref/forcerunginfalseread' '.html']);
      mask DialogControl PLCBlockTitle Prompt: Force Rung-In False Read
      mask Display: disp('_Force_RungIn_False');
  NOT : Logic  Operator=NOT  IconShape=distinctive  AllPortsSameDT=off  OutDataTypeStr=boolean
  Out1 : Outport  VectorParamsAs1DForOutWhenUnconnected=off
  wires:
  AND/1 -> Out1/1
  In1/1 -> AND/2
  ForceRungInFalseRead/1(Out1) -> NOT/1
  NOT/1 -> AND/1

== system elevatorMod/PLCControllerSuite/__Logic/Task/Program/__Logic/XIC48/__CoreVarRead ==
  DataRead : DataStoreRead  DataStoreName=xxx_PLC_VAR_F2UpDownBHold
  y : Outport  VectorParamsAs1DForOutWhenUnconnected=off
  wires:
  DataRead/1 -> y/1

== system elevatorMod/PLCControllerSuite/__Logic/Task/Program/__Logic/XIC49/BlockEnableRead ==
  __CoreLabelRead : Subsystem  Tag=CoreVarReadBlock  DisableCoverage=on  TreatAsAtomicUnit=on  mask{PLCBlockType=CoreLabelRead}
      mask init:
      | slplc.callbacks.initRoutineLabelRead(gcb);
      mask Help: web([docroot '/plccoder/ref/__corelabelread' '.html']);
      mask DialogControl PLCBlockTitle Prompt: Core Label Read
  Out1 : Outport  VectorParamsAs1DForOutWhenUnconnected=off
  wires:
  __CoreLabelRead/1(Out1) -> Out1/1

== system elevatorMod/PLCControllerSuite/__Logic/Task/Program/__Logic/XIC49/Instruction_Enable ==
  Rung-condition-in : Inport  OutDataTypeStr=BOOL
  Enable : EnablePort
  Logical Operator : Logic  OutDataTypeStr=BOOL
  __CoreVarRead : Subsystem  Tag=CoreVarReadBlock  DisableCoverage=on  TreatAsAtomicUnit=on  mask{PLCBlockType=CoreVarRead}
      mask init:
      | slplc.callbacks.initCoreVariable(gcb, 'read');
      mask Help: web([docroot '/plccoder/ref/__corevarread' '.html']);
      mask DialogControl PLCBlockTitle Prompt: Core Variable Read
  Rung-condition-out : Outport  VectorParamsAs1DForOutWhenUnconnected=off
  wires:
  __CoreVarRead/1(y) -> Logical Operator/2  "DataBit"
  Logical Operator/1 -> Rung-condition-out/1  "Rung-condition-out"
  Rung-condition-in/1 -> Logical Operator/1  "Rung-condition-in"

== system elevatorMod/PLCControllerSuite/__Logic/Task/Program/__Logic/XIC49/RungInOverride ==
  In1 : Inport
  AND : Logic  AllPortsSameDT=off  OutDataTypeStr=boolean
  ForceRungInFalseRead : Subsystem  DisableCoverage=on  TreatAsAtomicUnit=on  mask{PLCLabelTag=_Force_RungIn_False, PLCBlockType=ForceRungInFalseRead}
      mask prompts: PLCLabelTag "Label Tag:"
      mask init:
      | block = gcb;
      | maskObj = Simulink.Mask.get(block);
      | maskObj.Display = sprintf('disp(''%s'');', PLCLabelTag);
      mask Help: web([docroot '/plccoder/ref/forcerunginfalseread' '.html']);
      mask DialogControl PLCBlockTitle Prompt: Force Rung-In False Read
      mask Display: disp('_Force_RungIn_False');
  NOT : Logic  Operator=NOT  IconShape=distinctive  AllPortsSameDT=off  OutDataTypeStr=boolean
  Out1 : Outport  VectorParamsAs1DForOutWhenUnconnected=off
  wires:
  NOT/1 -> AND/1
  ForceRungInFalseRead/1(Out1) -> NOT/1
  In1/1 -> AND/2
  AND/1 -> Out1/1

== system elevatorMod/PLCControllerSuite/__Logic/Task/Program/__Logic/XIC49/__CoreVarRead ==
  DataRead : DataStoreRead  DataStoreName=xxx_PLC_VAR_S3L
  y : Outport  VectorParamsAs1DForOutWhenUnconnected=off
  wires:
  DataRead/1 -> y/1

== system elevatorMod/PLCControllerSuite/__Logic/Task/Program/__Logic/XIC5/BlockEnableRead ==
  __CoreLabelRead : Subsystem  Tag=CoreVarReadBlock  DisableCoverage=on  TreatAsAtomicUnit=on  mask{PLCBlockType=CoreLabelRead}
      mask init:
      | slplc.callbacks.initRoutineLabelRead(gcb);
      mask Help: web([docroot '/plccoder/ref/__corelabelread' '.html']);
      mask DialogControl PLCBlockTitle Prompt: Core Label Read
  Out1 : Outport  VectorParamsAs1DForOutWhenUnconnected=off
  wires:
  __CoreLabelRead/1(Out1) -> Out1/1

== system elevatorMod/PLCControllerSuite/__Logic/Task/Program/__Logic/XIC5/Instruction_Enable ==
  Rung-condition-in : Inport  OutDataTypeStr=BOOL
  Enable : EnablePort
  Logical Operator : Logic  OutDataTypeStr=BOOL
  __CoreVarRead : Subsystem  Tag=CoreVarReadBlock  DisableCoverage=on  TreatAsAtomicUnit=on  mask{PLCBlockType=CoreVarRead}
      mask init:
      | slplc.callbacks.initCoreVariable(gcb, 'read');
      mask Help: web([docroot '/plccoder/ref/__corevarread' '.html']);
      mask DialogControl PLCBlockTitle Prompt: Core Variable Read
  Rung-condition-out : Outport  VectorParamsAs1DForOutWhenUnconnected=off
  wires:
  Rung-condition-in/1 -> Logical Operator/1  "Rung-condition-in"
  Logical Operator/1 -> Rung-condition-out/1  "Rung-condition-out"
  __CoreVarRead/1(y) -> Logical Operator/2  "DataBit"

== system elevatorMod/PLCControllerSuite/__Logic/Task/Program/__Logic/XIC5/RungInOverride ==
  In1 : Inport
  AND : Logic  AllPortsSameDT=off  OutDataTypeStr=boolean
  ForceRungInFalseRead : Subsystem  DisableCoverage=on  TreatAsAtomicUnit=on  mask{PLCLabelTag=_Force_RungIn_False, PLCBlockType=ForceRungInFalseRead}
      mask prompts: PLCLabelTag "Label Tag:"
      mask init:
      | block = gcb;
      | maskObj = Simulink.Mask.get(block);
      | maskObj.Display = sprintf('disp(''%s'');', PLCLabelTag);
      mask Help: web([docroot '/plccoder/ref/forcerunginfalseread' '.html']);
      mask DialogControl PLCBlockTitle Prompt: Force Rung-In False Read
      mask Display: disp('_Force_RungIn_False');
  NOT : Logic  Operator=NOT  IconShape=distinctive  AllPortsSameDT=off  OutDataTypeStr=boolean
  Out1 : Outport  VectorParamsAs1DForOutWhenUnconnected=off
  wires:
  AND/1 -> Out1/1
  In1/1 -> AND/2
  ForceRungInFalseRead/1(Out1) -> NOT/1
  NOT/1 -> AND/1

== system elevatorMod/PLCControllerSuite/__Logic/Task/Program/__Logic/XIC5/__CoreVarRead ==
  DataRead : DataStoreRead  DataStoreName=xxx_PLC_VAR_StartHold
  y : Outport  VectorParamsAs1DForOutWhenUnconnected=off
  wires:
  DataRead/1 -> y/1

== system elevatorMod/PLCControllerSuite/__Logic/Task/Program/__Logic/XIC50/BlockEnableRead ==
  __CoreLabelRead : Subsystem  Tag=CoreVarReadBlock  DisableCoverage=on  TreatAsAtomicUnit=on  mask{PLCBlockType=CoreLabelRead}
      mask init:
      | slplc.callbacks.initRoutineLabelRead(gcb);
      mask Help: web([docroot '/plccoder/ref/__corelabelread' '.html']);
      mask DialogControl PLCBlockTitle Prompt: Core Label Read
  Out1 : Outport  VectorParamsAs1DForOutWhenUnconnected=off
  wires:
  __CoreLabelRead/1(Out1) -> Out1/1

== system elevatorMod/PLCControllerSuite/__Logic/Task/Program/__Logic/XIC50/Instruction_Enable ==
  Rung-condition-in : Inport  OutDataTypeStr=BOOL
  Enable : EnablePort
  Logical Operator : Logic  OutDataTypeStr=BOOL
  __CoreVarRead : Subsystem  Tag=CoreVarReadBlock  DisableCoverage=on  TreatAsAtomicUnit=on  mask{PLCBlockType=CoreVarRead}
      mask init:
      | slplc.callbacks.initCoreVariable(gcb, 'read');
      mask Help: web([docroot '/plccoder/ref/__corevarread' '.html']);
      mask DialogControl PLCBlockTitle Prompt: Core Variable Read
  Rung-condition-out : Outport  VectorParamsAs1DForOutWhenUnconnected=off
  wires:
  Rung-condition-in/1 -> Logical Operator/1  "Rung-condition-in"
  Logical Operator/1 -> Rung-condition-out/1  "Rung-condition-out"
  __CoreVarRead/1(y) -> Logical Operator/2  "DataBit"

== system elevatorMod/PLCControllerSuite/__Logic/Task/Program/__Logic/XIC50/RungInOverride ==
  In1 : Inport
  AND : Logic  AllPortsSameDT=off  OutDataTypeStr=boolean
  ForceRungInFalseRead : Subsystem  DisableCoverage=on  TreatAsAtomicUnit=on  mask{PLCLabelTag=_Force_RungIn_False, PLCBlockType=ForceRungInFalseRead}
      mask prompts: PLCLabelTag "Label Tag:"
      mask init:
      | block = gcb;
      | maskObj = Simulink.Mask.get(block);
      | maskObj.Display = sprintf('disp(''%s'');', PLCLabelTag);
      mask Help: web([docroot '/plccoder/ref/forcerunginfalseread' '.html']);
      mask DialogControl PLCBlockTitle Prompt: Force Rung-In False Read
      mask Display: disp('_Force_RungIn_False');
  NOT : Logic  Operator=NOT  IconShape=distinctive  AllPortsSameDT=off  OutDataTypeStr=boolean
  Out1 : Outport  VectorParamsAs1DForOutWhenUnconnected=off
  wires:
  AND/1 -> Out1/1
  In1/1 -> AND/2
  ForceRungInFalseRead/1(Out1) -> NOT/1
  NOT/1 -> AND/1

== system elevatorMod/PLCControllerSuite/__Logic/Task/Program/__Logic/XIC50/__CoreVarRead ==
  DataRead : DataStoreRead  DataStoreName=xxx_PLC_VAR_S2H
  y : Outport  VectorParamsAs1DForOutWhenUnconnected=off
  wires:
  DataRead/1 -> y/1

== system elevatorMod/PLCControllerSuite/__Logic/Task/Program/__Logic/XIC51/BlockEnableRead ==
  __CoreLabelRead : Subsystem  Tag=CoreVarReadBlock  DisableCoverage=on  TreatAsAtomicUnit=on  mask{PLCBlockType=CoreLabelRead}
      mask init:
      | slplc.callbacks.initRoutineLabelRead(gcb);
      mask Help: web([docroot '/plccoder/ref/__corelabelread' '.html']);
      mask DialogControl PLCBlockTitle Prompt: Core Label Read
  Out1 : Outport  VectorParamsAs1DForOutWhenUnconnected=off
  wires:
  __CoreLabelRead/1(Out1) -> Out1/1

== system elevatorMod/PLCControllerSuite/__Logic/Task/Program/__Logic/XIC51/Instruction_Enable ==
  Rung-condition-in : Inport  OutDataTypeStr=BOOL
  Enable : EnablePort
  Logical Operator : Logic  OutDataTypeStr=BOOL
  __CoreVarRead : Subsystem  Tag=CoreVarReadBlock  DisableCoverage=on  TreatAsAtomicUnit=on  mask{PLCBlockType=CoreVarRead}
      mask init:
      | slplc.callbacks.initCoreVariable(gcb, 'read');
      mask Help: web([docroot '/plccoder/ref/__corevarread' '.html']);
      mask DialogControl PLCBlockTitle Prompt: Core Variable Read
  Rung-condition-out : Outport  VectorParamsAs1DForOutWhenUnconnected=off
  wires:
  Rung-condition-in/1 -> Logical Operator/1  "Rung-condition-in"
  Logical Operator/1 -> Rung-condition-out/1  "Rung-condition-out"
  __CoreVarRead/1(y) -> Logical Operator/2  "DataBit"

== system elevatorMod/PLCControllerSuite/__Logic/Task/Program/__Logic/XIC51/RungInOverride ==
  In1 : Inport
  AND : Logic  AllPortsSameDT=off  OutDataTypeStr=boolean
  ForceRungInFalseRead : Subsystem  DisableCoverage=on  TreatAsAtomicUnit=on  mask{PLCLabelTag=_Force_RungIn_False, PLCBlockType=ForceRungInFalseRead}
      mask prompts: PLCLabelTag "Label Tag:"
      mask init:
      | block = gcb;
      | maskObj = Simulink.Mask.get(block);
      | maskObj.Display = sprintf('disp(''%s'');', PLCLabelTag);
      mask Help: web([docroot '/plccoder/ref/forcerunginfalseread' '.html']);
      mask DialogControl PLCBlockTitle Prompt: Force Rung-In False Read
      mask Display: disp('_Force_RungIn_False');
  NOT : Logic  Operator=NOT  IconShape=distinctive  AllPortsSameDT=off  OutDataTypeStr=boolean
  Out1 : Outport  VectorParamsAs1DForOutWhenUnconnected=off
  wires:
  AND/1 -> Out1/1
  In1/1 -> AND/2
  ForceRungInFalseRead/1(Out1) -> NOT/1
  NOT/1 -> AND/1

== system elevatorMod/PLCControllerSuite/__Logic/Task/Program/__Logic/XIC51/__CoreVarRead ==
  DataRead : DataStoreRead  DataStoreName=xxx_PLC_VAR_F1PBHold
  y : Outport  VectorParamsAs1DForOutWhenUnconnected=off
  wires:
  DataRead/1 -> y/1

== system elevatorMod/PLCControllerSuite/__Logic/Task/Program/__Logic/XIC52/BlockEnableRead ==
  __CoreLabelRead : Subsystem  Tag=CoreVarReadBlock  DisableCoverage=on  TreatAsAtomicUnit=on  mask{PLCBlockType=CoreLabelRead}
      mask init:
      | slplc.callbacks.initRoutineLabelRead(gcb);
      mask Help: web([docroot '/plccoder/ref/__corelabelread' '.html']);
      mask DialogControl PLCBlockTitle Prompt: Core Label Read
  Out1 : Outport  VectorParamsAs1DForOutWhenUnconnected=off
  wires:
  __CoreLabelRead/1(Out1) -> Out1/1

== system elevatorMod/PLCControllerSuite/__Logic/Task/Program/__Logic/XIC52/Instruction_Enable ==
  Rung-condition-in : Inport  OutDataTypeStr=BOOL
  Enable : EnablePort
  Logical Operator : Logic  OutDataTypeStr=BOOL
  __CoreVarRead : Subsystem  Tag=CoreVarReadBlock  DisableCoverage=on  TreatAsAtomicUnit=on  mask{PLCBlockType=CoreVarRead}
      mask init:
      | slplc.callbacks.initCoreVariable(gcb, 'read');
      mask Help: web([docroot '/plccoder/ref/__corevarread' '.html']);
      mask DialogControl PLCBlockTitle Prompt: Core Variable Read
  Rung-condition-out : Outport  VectorParamsAs1DForOutWhenUnconnected=off
  wires:
  __CoreVarRead/1(y) -> Logical Operator/2  "DataBit"
  Logical Operator/1 -> Rung-condition-out/1  "Rung-condition-out"
  Rung-condition-in/1 -> Logical Operator/1  "Rung-condition-in"
